simulink model "main_system"  (R2022b)
settings: Solver=VariableStepAuto  StartTime=0.0  StopTime=10.0  RelTol=1e-3
settings Model: Creator=LeonK  LastModifiedBy=LeonK

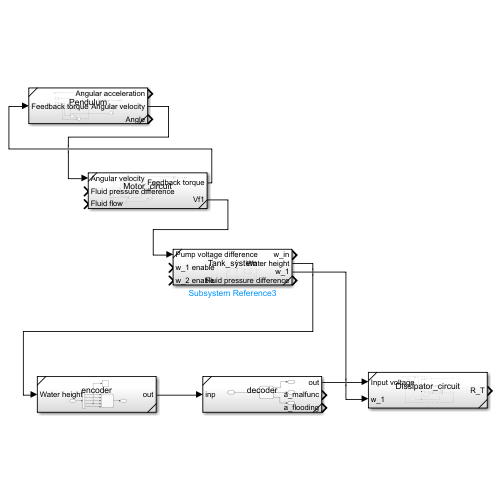
[thumbnail: Simulink's stored preview of the top-level diagram]
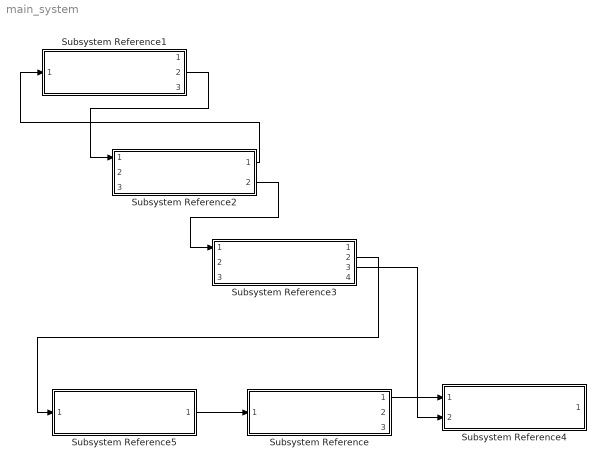
== system main_system ==
  Subsystem Reference : Subsystem  ReferencedSubsystem=decoder
  Subsystem Reference1 : Subsystem  ReferencedSubsystem=Pendulum
  Subsystem Reference2 : Subsystem  ReferencedSubsystem=Motor_circuit
  Subsystem Reference3 : Subsystem  ReferencedSubsystem=Tank_system
  Subsystem Reference4 : Subsystem  ReferencedSubsystem=Dissipator_circuit
  Subsystem Reference5 : Subsystem  ReferencedSubsystem=encoder
  wires:
  Subsystem Reference2/1 -> Subsystem Reference1/1
  Subsystem Reference1/2 -> Subsystem Reference2/1
  Subsystem Reference/1 -> Subsystem Reference4/1
  Subsystem Reference5/1 -> Subsystem Reference/1
  Subsystem Reference3/2 -> Subsystem Reference5/1
  Subsystem Reference2/2 -> Subsystem Reference3/1
  Subsystem Reference3/3 -> Subsystem Reference4/2
